simulink model "single_phase_pv_inverter_c2000"  (Simulink 7.3)
settings: Solver=ode45  StartTime=0.0  StopTime=4  RelTol=1e-3
InitFcn:
  | % Processor selection for I/O assignment
  | % The chosen Target in the Coder Options window must match the selected MCU.
  | % Set the variable 'type_evm' to the following strings to choose a specific target:
  | 
  |   type_evm = 'TI28069';    % TI28069 Piccolo Launchpad
  | % type_evm = 'TI28377S';   % TI28377S Delfino Launchpad
  | % type_evm = 'TI28379LP';  % TI28379D Delfino Launchpad
  | % type_evm = 'TI280049C';  % TI280049C Piccolo Launchpad
  | % type_evm = 'TI28379CC';  % TI28379D Delfino Controlcard
  | % type_evm = 'TI28388D';   % TI28388D Controlcard
  | 
  | % Configure I/O based on processor
  | switch (type_evm)
  | 	case 'TI28069'
  | 	% Configuration for TI28069 Launchpad
  | 	%on the Plant side
  | 		AO_RTBox_DC = [0:1];
  | 		AO_RTBox_AC = [2:3];
  | 		PWMCAP_RTBox_sw = [0:3];
  | 		DO_RTBox_En = 4;
  | 		DI_RTBox_Power = 22;
  | 		AO_Vmax = 3.3;
  | 		AO_Factor = 1;
  | 
  | 	%on the Controller side
  | 		ADC_DSP_ADC = [7,1+8,2,2+8];
  | 		PWM_DSP_PWM = [1,2];
  | 		DO_DSP_LED = 34;
  | 		DI_DSP_En = 13;
  | 		PWR_DSP_GPIO = 27;
  | 		SCI_DSP = [28, 29];
  | 		ADC_Vmax = 3.3;
  | 
  | 	case 'TI28377S'
  | 	% Configuration for TI28377S Launchpad
  | 	%on the Plant side
  | 		AO_RTBox_DC = [6,10];
  | 		AO_RTBox_AC = [12,14];
  | 		PWMCAP_RTBox_sw = 2:5;
  | 		DO_RTBox_En = 6;
  | 		DI_RTBox_Power = 26;
  | 		AO_Vmax = 3.3;
  | 		AO_Factor = 1;
  | 
  | 	%on the Controller side
  | 		ADC_DSP_ADC = [1,5,3,4];
  | 		PWM_DSP_PWM = [8,9];
  | 		DO_DSP_LED = 12;
  | 		DI_DSP_En = 72;
  | 		PWR_DSP_GPIO = 43;
  | 		SCI_DSP = [85, 84];
  | 		ADC_Vmax = 3.3;
  | 
  | 	case 'TI28379LP'
  | 	% Configuration for TI28379D Launchpad
  | 	%on the Plant side
  | 		AO_RTBox_DC = [0,3];
  | 		AO_RTBox_AC = [11,14];
  | 		PWMCAP_RTBox_sw = 0:3;
  | 		DO_RTBox_En = 6;
  | 		DI_RTBox_Power = 22;
  | 		AO_Vmax = 3.3;
  | 		AO_Factor = 1;
  | 
  | 	%on the Controller side
  | 		ADC_DSP_ADC = [14,3,5,4];
  | 		PWM_DSP_PWM = [1,2];
  | 		DO_DSP_LED = 34;
  | 		DI_DSP_En = 124;
  | 		PWR_DSP_GPIO = 66;
  | 		SCI_DSP = [43, 42];
  | 		ADC_Vmax = 3.3;
  | 
  | 	case 'TI280049C'
  | 	% Configuration for TI280049C Launchpad
  | 	%on the Plant side
  | 		AO_RTBox_DC = [0,6];
  | 		AO_RTBox_AC = [8,14];
  | 		PWMCAP_RTBox_sw = 0:3;
  | 		DO_RTBox_En = 4;
  | 		DI_RTBox_Power = 24;
  | 		AO_Vmax = 3.3;
  | 		AO_Factor = 1;
  | 
  | 	%on the Controller side
  | 		ADC_DSP_ADC = [5,9,6,3];
  | 		PWM_DSP_PWM = [6,5];
  | 		DO_DSP_LED = 34;
  | 		DI_DSP_En = 58;
  | 		PWR_DSP_GPIO = 56;
  | 		SCI_DSP = [28, 29];
  | 		ADC_Vmax = 3.3;
  | 
  | 		case 'TI28379CC'
  | 	% Configuration for TI28379D Controlcard
  | 	%on the Plant side
  | 		AO_RTBox_DC = [15 ,13];
  | 		AO_RTBox_AC = [11, 9];
  | 		PWMCAP_RTBox_sw = 0:3;
  | 		DO_RTBox_En = 21;
  | 		DI_RTBox_Power = 14;
  | 		AO_Vmax = 5.0;
  | 		AO_Factor = 1.54; % breakout board scaling 6.8k/4.42k
  | 
  | 	%on the Controller side
  | 		ADC_DSP_ADC = [0,1,2,3];
  | 		PWM_DSP_PWM = [1,2];
  | 		DO_DSP_LED = 34;
  | 		DI_DSP_En = 40;
  | 		PWR_DSP_GPIO = 39;
  | 		SCI_DSP = [28, 29];
  | 		ADC_Vmax = 3.0;
  | 
  | 		case 'TI28388D'
  | 	% Configuration for TI28388D Controlcard
  | 	%on the Plant side
  | 		AO_RTBox_DC = [15 ,13];
  | 		AO_RTBox_AC = [11, 9];
  | 		PWMCAP_RTBox_sw = 0:3;
  | 		DO_RTBox_En = 21;
  | 		DI_RTBox_Power = 14;
  | 		AO_Vmax = 5.0;
  | 		AO_Factor = 1.54; % breakout board scaling 6.8k/4.42k
  | 
  | 	%on the Controller side
  | 		ADC_DSP_ADC = [0,1,2,3];
  | 		PWM_DSP_PWM = [1,2];
  | 		DO_DSP_LED = 34;
  | 		DI_DSP_En = 40;
  | 		PWR_DSP_GPIO = 39;
  | 		SCI_DSP = [28, 29];
  | 		ADC_Vmax = 3.0;
  | 
  | 	otherwise
  | 	error('Unknown evaluation module selection, please choose either ''TI28069'', ''TI28377S'', ''TI28379LP'', ''TI280049C'', ''TI28379CC'' or ''TI28388D''.')
  | end
  | 
  | % switching frequency
  | fs=(25e3)/2 % switching frequency in Hz
  | 
  | % controller dicretizaton
  | fc=25e3; % sample rate of the controller subsystem (Base task) in Hz
  | Ts_controller=1/fc; % sample step size of the Base task in sec
  | Ts_MPP = 2.2e-3; %sample step size of the MPP task in sec
  | Ts_Volt= 4e-4; %sample step size of the voltage controller task in sec
  | Ts_LED = 0.1;  %sample step size of the LED task in sec
  | 
  | % plant dicretizaton
  | Ts_plant = 1/fc/16; % sample step size of the plant subsystem in sec
  | 
  | 
  | % system parameters
  | Prated=3000; % Rated power in W
  | Vdc0=380;
  | Idc0=Prated/Vdc0;
  | Iacmax=40;
  | Vgrid = 325;
  | Fgrid = 50;
  | 
  | % scaling
  | Vdc_scl = ADC_Vmax/(2*Vdc0);
  | Idc_scl = ADC_Vmax/(2*Idc0);
  | 
  | Vg_scl = ADC_Vmax/(4*Vgrid);
  | Vg_ofs = ADC_Vmax/2;
  | 
  | Ig_scl = ADC_Vmax/(2*Iacmax);
  | Ig_ofs = ADC_Vmax/2;
undefined symbols (not defined in the file): plecs
settings Model: Creator=kris  LastModifiedBy=manaswini  ExtModeTrigMode=oneshot  ExtModeArmWhenConnect=off  ExtModeAutoUpdateStatusClock=off
settings DataIOCC: LimitDataPoints=off  ReturnWorkspaceOutputs=off  SignalLoggingName=sigsOut
settings OptimizationCC: BooleanDataType=off  ExpressionDepthLimit=128  InitFltsAndDblsToZero=on
settings DebuggingCC: SaveWithParameterizedLinksMsg=none  SignalResolutionControl=TryResolveAllWithWarning  SolverPrmCheckMsg=none  MultiTaskDSMMsg=warning  MultiTaskCondExecSysMsg=none  FcnCallInpInsideContextMsg=Enable All  StrictBusMsg=ErrorLevel1
settings HardwareCC: TargetHWDeviceType=32-bit Generic  TargetUnknown=on  ProdEqTarget=off
settings RTWCC: IncludeERTFirstTime=on
settings CodeAppCC: CustomSymbolStrType=$N$R$M_T
settings GRTTargetCC: TargetFcnLib=ansi_tfl_tmw.mat  TargetFunctionLibrary=C89/C90 (ANSI)  ModelReferenceCompliant=off

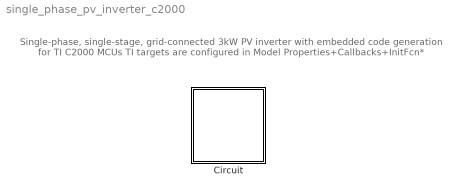
== system single_phase_pv_inverter_c2000 ==
  note: Single-phase, single-stage, grid-connected 3kW PV inverter
      | with embedded code generation for TI C2000 MCUs
      | TI targets are configured in Model Properties+Callbacks+InitFcn*
  Circuit : Subsystem  LoadFcn=plecs('sl', 200);  InitFcn=plecs('sl', 214);  StartFcn=plecs('sl', 208);  StopFcn=plecs('sl', 209);  ClipboardFcn=plecs('sl', 212, 26);  mask(PlecsCircuit){PLECSData=<binary blob, 23116 chars, not shown>}
      mask prompts: PLECSData "PLECS Data (Do not delete or modify!)"
      mask help: Drag this block into a Simulink model to create a new electrical circuit.
      mask init:
      | % PLACE CUSTOM INITIALIZATIONS ABOVE
      | % DO NOT REMOVE
      | plecs('sl', 215);
      | % DO NOT REMOVE
      settings: CopyFcn=plecs('sl', 203);  DeleteFcn=plecs('sl', 205);  UndoDeleteFcn=plecs('sl', 206);  PreSaveFcn=plecs('sl', 211);  PostSaveFcn=plecs('sl', 201);  NameChangeFcn=plecs('sl', 210);  DestroyFcn=plecs('sl', 207);  PreCopyFcn=plecs('sl', 216);  OpenFcn=plecs('sl', 202);  ErrorFcn=plerrorfcn
      mask Display: disp('PLECS\nCircuit')

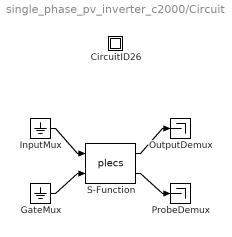
== system single_phase_pv_inverter_c2000/Circuit ==
  " CircuitID26 " : Subsystem
  " GateMux " : Ground
  " InputMux " : Ground
  " OutputDemux " : Terminator
  " ProbeDemux " : Terminator
  " S-Function " : S-Function  FunctionName=plecs  EnableBusSupport=off
  wires:
  " InputMux "/1 -> " S-Function "/1
  " GateMux "/1 -> " S-Function "/2
  " S-Function "/1 -> " OutputDemux "/1
  " S-Function "/2 -> " ProbeDemux "/1

== system single_phase_pv_inverter_c2000/Circuit/ CircuitID26  ==
